simulink model "a2DOF"  (R2021a)
settings: Solver=VariableStepAuto  StartTime=0.0  StopTime=20  RelTol=1e-3
undefined symbols (not defined in the file): Caf, Car, Iz, Lf, Lr, m
settings Model: Creator=RickyFang  LastModifiedBy=RickyFang

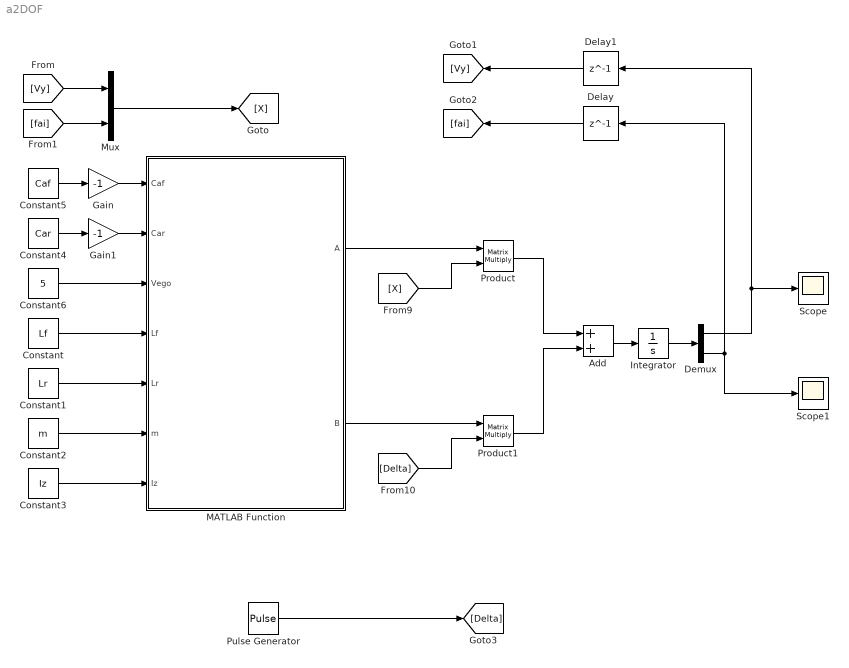
== system a2DOF ==
  Add : Sum
  Constant : Constant  Value=Lf
  Constant1 : Constant  Value=Lr
  Constant2 : Constant  Value=m
  Constant3 : Constant  Value=Iz
  Constant4 : Constant  Value=Car
  Constant5 : Constant  Value=Caf
  Constant6 : Constant  Value=5
  Delay : Delay  DelayLength=1
  Delay1 : Delay  DelayLength=1
  Demux : Demux  Outputs=2
  Gain : Gain  Gain=-1
  Gain1 : Gain  Gain=-1
  Integrator : Integrator
  MATLAB Function : MATLAB Function  TreatAsAtomicUnit=on
  Mux : Mux  Inputs=2
  Product : Product  Multiplication=Matrix(*)
  Product1 : Product  Multiplication=Matrix(*)
  Pulse Generator : DiscretePulseGenerator  PulseType=Time based  Amplitude=0.1  Period=1  PulseWidth=0.1
  Scope : Scope
  Scope1 : Scope
  wires:
  [fai] -> Mux/2
  [Vy] -> Mux/1
  Mux/1 -> [X]
  Constant3/1 -> MATLAB Function/7(Iz)
  Constant/1 -> MATLAB Function/4(Lf)
  Constant1/1 -> MATLAB Function/5(Lr)
  Constant2/1 -> MATLAB Function/6(m)
  Constant6/1 -> MATLAB Function/3(Vego)
  Constant4/1 -> Gain1/1
  Constant5/1 -> Gain/1
  MATLAB Function/1(A) -> Product/1
  [X] -> Product/2
  MATLAB Function/2(B) -> Product1/1
  [Delta] -> Product1/2
  Product/1 -> Add/1
  Product1/1 -> Add/2
  Add/1 -> Integrator/1
  Demux/1 -> Delay1/1, Scope/1
  Demux/2 -> Delay/1, Scope1/1
  Integrator/1 -> Demux/1
  Delay1/1 -> [Vy]
  Delay/1 -> [fai]
  Pulse Generator/1 -> [Delta]
  Gain/1 -> MATLAB Function/1(Caf)
  Gain1/1 -> MATLAB Function/2(Car)

== matlab function a2DOF/MATLAB Function ==
  data: Caf input; A output; Car input; Vego input; Lf input; Lr input; m input; Iz input; B output
function [A,B] = fun_2DoF(Caf,Car,Vego,Lf,Lr,m,Iz)

A = [-(2*Caf+2*Car)/(m*Vego) -Vego-(2*Caf*Lf-2*Car*Lr)/(m*Vego);
     -(2*Caf*Lf-2*Car*Lr)/(Iz*Vego) -(2*Caf*Lf*Lf+2*Car*Lr*Lr)/(Iz*Vego)];

B = [2*Caf/m;2*Caf*Lf/Iz];
